simulink model "compare_filters"  (R2025a)
settings: Solver=VariableStepAuto  StartTime=0.0  StopTime=1.5  RelTol=1e-3
values from neighbouring files (symbols this model uses):
  phi_corr_LUT_param = Simulink.Parameter(phi_corr_LUT)    [lut_script.m]
undefined symbols (not defined in the file or in its folder): closed_loop, D_duty_cycle, D_m, DiscIntNeverNeededParam, hall_errors, I_duty_cycle, J_t, L_ss, lambda_m, P, P_duty_cycle, r_s, R_vs, T_m, theta_v, use_LUT, V_bus
libraries: spsMosfetLib x18, spsSeriesRLCBranchLib x12, spsVoltageMeasurementLib x9, spsControlledCurrentSourceLib x9, slpidlib x6, eeGeneralControl x3, simulink x3, embmathops x3, spsControlledVoltageSourceLib x3, spsPWMGeneratorDCDCLib x3, spsDCVoltageSourceLib x3, sps_lib x3
(part 1 of 3)
settings Model: Creator=rnashota.stu  LastModifiedBy=rnashota.stu

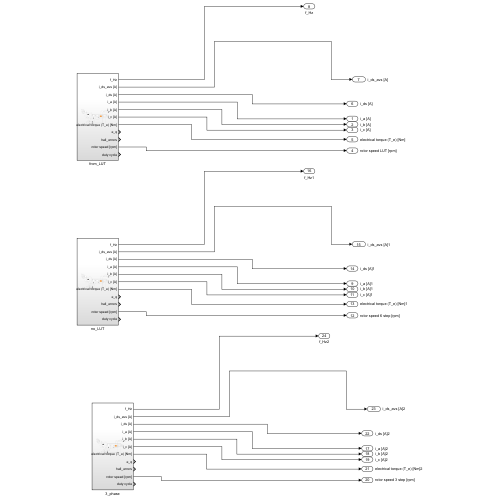
[thumbnail: Simulink's stored preview of the top-level diagram]
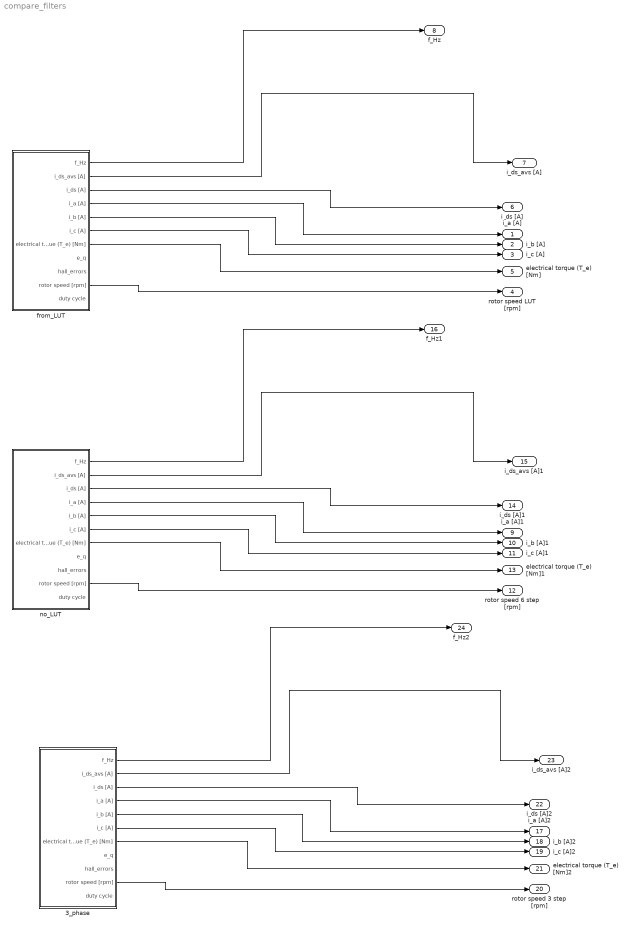
== system compare_filters ==
  3_phase : Subsystem
  from_LUT : Subsystem
  no_LUT : Subsystem
  i_a [A] : Outport
  i_b [A] : Outport  Port=2
  i_c [A] : Outport  Port=3
  rotor speed LUT [rpm] : Outport  Port=4
  electrical torque (T_e) [Nm] : Outport  Port=5
  i_ds [A] : Outport  Port=6
  i_ds_avs [A] : Outport  Port=7
  f_Hz : Outport  Port=8
  i_a [A]1 : Outport  Port=9
  i_b [A]1 : Outport  Port=10
  i_c [A]1 : Outport  Port=11
  rotor speed 6 step [rpm] : Outport  Port=12
  electrical torque (T_e) [Nm]1 : Outport  Port=13
  i_ds [A]1 : Outport  Port=14
  i_ds_avs [A]1 : Outport  Port=15
  f_Hz1 : Outport  Port=16
  i_a [A]2 : Outport  Port=17
  i_b [A]2 : Outport  Port=18
  i_c [A]2 : Outport  Port=19
  rotor speed 3 step [rpm] : Outport  Port=20
  electrical torque (T_e) [Nm]2 : Outport  Port=21
  i_ds [A]2 : Outport  Port=22
  i_ds_avs [A]2 : Outport  Port=23
  f_Hz2 : Outport  Port=24
  wires:
  from_LUT/1(f_Hz) -> f_Hz/1
  from_LUT/2(i_ds_avs [A]) -> i_ds_avs [A]/1
  from_LUT/3(i_ds [A]) -> i_ds [A]/1
  from_LUT/4(i_a [A]) -> i_a [A]/1
  from_LUT/5(i_b [A]) -> i_b [A]/1
  from_LUT/6(i_c [A]) -> i_c [A]/1
  from_LUT/7(electrical torque (T_e) [Nm]) -> electrical torque (T_e) [Nm]/1
  from_LUT/10(rotor speed [rpm]) -> rotor speed LUT [rpm]/1
  no_LUT/7(electrical torque (T_e) [Nm]) -> electrical torque (T_e) [Nm]1/1
  no_LUT/10(rotor speed [rpm]) -> rotor speed 6 step [rpm]/1
  no_LUT/2(i_ds_avs [A]) -> i_ds_avs [A]1/1
  no_LUT/3(i_ds [A]) -> i_ds [A]1/1
  no_LUT/6(i_c [A]) -> i_c [A]1/1
  no_LUT/1(f_Hz) -> f_Hz1/1
  no_LUT/4(i_a [A]) -> i_a [A]1/1
  no_LUT/5(i_b [A]) -> i_b [A]1/1
  3_phase/3(i_ds [A]) -> i_ds [A]2/1
  3_phase/5(i_b [A]) -> i_b [A]2/1
  3_phase/2(i_ds_avs [A]) -> i_ds_avs [A]2/1
  3_phase/6(i_c [A]) -> i_c [A]2/1
  3_phase/10(rotor speed [rpm]) -> rotor speed 3 step [rpm]/1
  3_phase/4(i_a [A]) -> i_a [A]2/1
  3_phase/1(f_Hz) -> f_Hz2/1
  3_phase/7(electrical torque (T_e) [Nm]) -> electrical torque (T_e) [Nm]2/1

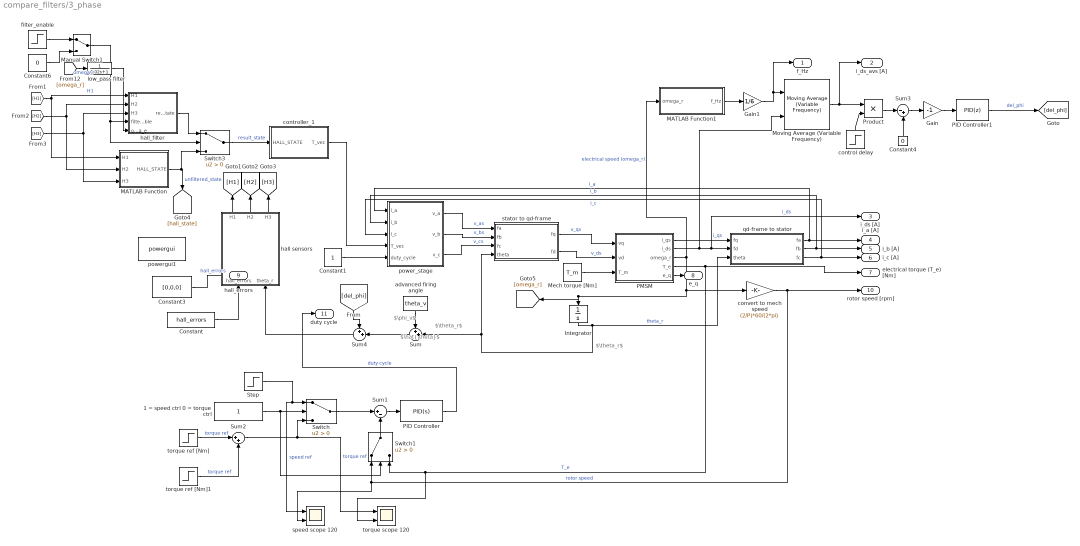
== system compare_filters/3_phase ==
  note: $\theta_r$
  note: $\hat{\theta}$
  note: $\phi_v$
  note: $\theta_r$
  1 = speed ctrl 0 = torque ctrl : Constant
  Constant : Constant  Value=hall_errors
  Constant1 : Constant
  Constant3 : Constant  Value=[0,0,0]
  Constant4 : Constant  Value=0
  Constant6 : Constant  Value=0
  Gain : Gain  Gain=-1
  Gain1 : Gain  Gain=1/6
  Integrator : Integrator
  MATLAB Function : MATLAB Function  TreatAsAtomicUnit=on
  MATLAB Function1 : MATLAB Function  TreatAsAtomicUnit=on
  Manual Switch1 : ManualSwitch
  Mech torque [Nm] : Constant  Value=T_m
  Moving Average (Variable Frequency) : eeGeneralControl/Moving Average (Variable Frequency)  VariantControl=Variant1  LabelModeActiveChoice=Continuous  f0=60  fmin=1  x0=0  BufferSize=32768  Ts=0
      settings: LibrarySourceBlock=|
      | ee_sl_lib/General Control/Moving Average
      | (Variable Frequency)
  PID Controller : slpidlib/PID Controller  Controller=PID  Form=Parallel  TimeDomain=Continuous-time  UseExternalTs=off  SampleTime=-1  IntegratorMethod=Forward Euler  FilterMethod=Forward Euler  ControllerParametersSource=internal  P=P_duty_cycle  I=I_duty_cycle  UseKiTs=off  D=D_duty_cycle  UseExternalDerivativeSource=off  N=100  UseFilter=on  TunerSelectOption=Transfer Function Based (PID Tuner App)  InitialConditionSource=internal  InitialConditionForIntegrator=0  InitialConditionForFilter=0  DifferentiatorICPrevScaledInput=0  ExternalReset=none  TrackingMode=off  Kt=1  LimitOutput=on  SatLimitsSource=internal  UpperSaturationLimit=1  LowerSaturationLimit=0  LinearizeAsGain=on  AntiWindupMode=none  Kb=1  LimitIntegrator=off  UpperIntegratorSaturationLimit=inf  LowerIntegratorSaturationLimit=-inf  POutMin=[]  POutMax=[]  IOutMin=[]  IOutMax=[]  DOutMin=[]  DOutMax=[]  NOutMin=[]  NOutMax=[]  SumOutMin=[]  SumOutMax=[]  SaturationOutMin=[]  SaturationOutMax=[]  PParamMin=[]  PParamMax=[]  IParamMin=[]  IParamMax=[]  DParamMin=[]  DParamMax=[]  NParamMin=[]  NParamMax=[]  KbParamMin=[]  KbParamMax=[]  KtParamMin=[]  KtParamMax=[]  KbOutMin=[]  KbOutMax=[]  KtOutMin=[]  KtOutMax=[]  IntegratorOutMin=[]  IntegratorOutMax=[]  FilterOutMin=[]  FilterOutMax=[]  SumI1OutMin=[]  SumI1OutMax=[]  SumI2OutMin=[]  SumI2OutMax=[]  SumI3OutMin=[]  SumI3OutMax=[]  SumI4OutMin=[]  SumI4OutMax=[]  SumDOutMin=[]  SumDOutMax=[]  DifferentiatorOutMin=[]  DifferentiatorOutMax=[]  FilterDiffOutCoefMin=[]  FilterDiffOutCoefMax=[]  ReciprocalOutMin=[]  ReciprocalOutMax=[]  SumDenOutMin=[]  SumDenOutMax=[]  SumNumOutMin=[]  SumNumOutMax=[]  DivideOutMin=[]  DivideOutMax=[]  UdiffTsProdOutMin=[]  UdiffTsProdOutMax=[]  NTsProdOutMin=[]  NTsProdOutMax=[]  UintegralTsProdOutMin=[]  UintegralTsProdOutMax=[]  UngainTsProdOutMin=[]  UngainTsProdOutMax=[]  ClampingZeroOutDataTypeStr=Inherit: Inherit via back propagation  ClampingZeroOutMin=[]  ClampingZeroOutMax=[]  FilterDenConstantOutDataTypeStr=Inherit: Inherit via back propagation  FilterDenConstantOutMin=[]  FilterDenConstantOutMax=[]  PCopyOutDataTypeStr=Inherit: Inherit via back propagation  PCopyOutMin=[]  PCopyOutMax=[]  NCopyOutDataTypeStr=Inherit: Inherit via back propagation  NCopyOutMin=[]  NCopyOutMax=[]  IntegratorContinuousStateAttributes=''  IntegratorStateMustResolveToSignalObject=off  IntegratorRTWStateStorageClass=Auto  FilterContinuousStateAttributes=''  FilterStateMustResolveToSignalObject=off  FilterRTWStateStorageClass=Auto  ParallelPVariant=InternalParameters  IdealPVariant=Disabled  IVariant=InternalParameters  DVariant=InternalParameters  IntegratorVariant=Continuous  SatVariant=Enabled  AWVariant=Passthrough  PCopyVariant=Disabled  TRVariant=Disabled  FdbkBlocksVariant=Forward  IdealPFdbkVariant=Disabled  SatFdbkVariant=Disabled  DerivativeFilterVariant=ContFilter  NVariant=InternalParameters  NCopyVariant=Disabled  FilterICVariant=InternalICsFilter  IntegratorICVariant=InternalICs  ExternalResetVariant=Disabled  TRSumVariant=Passthrough  SumFdbkVariant=Disabled  SumVariant=Sum_PID  TsampFilterVariant=InternalTs  TsampNgainVariant=Passthrough  TsampIntegralVariant=Disabled_SignalSpec  ExternalSaturationOutDataTypeStr=Inherit: Same as second input  DerivativeSourceVariant=ErrorSignal  PreIntVariant=InternalPreInt
  PID Controller1 : slpidlib/PID Controller  Controller=PID  Form=Parallel  TimeDomain=Discrete-time  UseExternalTs=off  SampleTime=-1  IntegratorMethod=Forward Euler  FilterMethod=Forward Euler  ControllerParametersSource=internal  P=0.0068  I=0.744  UseKiTs=off  D=0  UseExternalDerivativeSource=off  N=100  UseFilter=on  TunerSelectOption=Transfer Function Based (PID Tuner App)  InitialConditionSource=internal  InitialConditionForIntegrator=0  InitialConditionForFilter=0  DifferentiatorICPrevScaledInput=0  ExternalReset=none  TrackingMode=off  Kt=1  LimitOutput=on  SatLimitsSource=internal  UpperSaturationLimit=pi/3  LowerSaturationLimit=-pi/3  LinearizeAsGain=on  AntiWindupMode=none  Kb=1  LimitIntegrator=off  UpperIntegratorSaturationLimit=inf  LowerIntegratorSaturationLimit=-inf  POutMin=[]  POutMax=[]  IOutMin=[]  IOutMax=[]  DOutMin=[]  DOutMax=[]  NOutMin=[]  NOutMax=[]  SumOutMin=[]  SumOutMax=[]  SaturationOutMin=[]  SaturationOutMax=[]  PParamMin=[]  PParamMax=[]  IParamMin=[]  IParamMax=[]  DParamMin=[]  DParamMax=[]  NParamMin=[]  NParamMax=[]  KbParamMin=[]  KbParamMax=[]  KtParamMin=[]  KtParamMax=[]  KbOutMin=[]  KbOutMax=[]  KtOutMin=[]  KtOutMax=[]  IntegratorOutMin=[]  IntegratorOutMax=[]  FilterOutMin=[]  FilterOutMax=[]  SumI1OutMin=[]  SumI1OutMax=[]  SumI2OutMin=[]  SumI2OutMax=[]  SumI3OutMin=[]  SumI3OutMax=[]  SumI4OutMin=[]  SumI4OutMax=[]  SumDOutMin=[]  SumDOutMax=[]  DifferentiatorOutMin=[]  DifferentiatorOutMax=[]  FilterDiffOutCoefMin=[]  FilterDiffOutCoefMax=[]  ReciprocalOutMin=[]  ReciprocalOutMax=[]  SumDenOutMin=[]  SumDenOutMax=[]  SumNumOutMin=[]  SumNumOutMax=[]  DivideOutMin=[]  DivideOutMax=[]  UdiffTsProdOutMin=[]  UdiffTsProdOutMax=[]  NTsProdOutMin=[]  NTsProdOutMax=[]  UintegralTsProdOutMin=[]  UintegralTsProdOutMax=[]  UngainTsProdOutMin=[]  UngainTsProdOutMax=[]  ClampingZeroOutDataTypeStr=Inherit: Inherit via back propagation  ClampingZeroOutMin=[]  ClampingZeroOutMax=[]  FilterDenConstantOutDataTypeStr=Inherit: Inherit via back propagation  FilterDenConstantOutMin=[]  FilterDenConstantOutMax=[]  PCopyOutDataTypeStr=Inherit: Inherit via back propagation  PCopyOutMin=[]  PCopyOutMax=[]  NCopyOutDataTypeStr=Inherit: Inherit via back propagation  NCopyOutMin=[]  NCopyOutMax=[]  IntegratorContinuousStateAttributes=''  IntegratorStateMustResolveToSignalObject=off  IntegratorRTWStateStorageClass=Auto  FilterContinuousStateAttributes=''  FilterStateMustResolveToSignalObject=off  FilterRTWStateStorageClass=Auto  ParallelPVariant=InternalParameters  IdealPVariant=Disabled  IVariant=InternalParameters  DVariant=InternalParameters  IntegratorVariant=Discrete  SatVariant=Enabled  AWVariant=Passthrough  PCopyVariant=Disabled  TRVariant=Disabled  FdbkBlocksVariant=Forward  IdealPFdbkVariant=Disabled  SatFdbkVariant=Disabled  DerivativeFilterVariant=ForwardEulerFilter  NVariant=InternalParameters  NCopyVariant=Disabled  FilterICVariant=InternalICsFilter  IntegratorICVariant=InternalICs  ExternalResetVariant=Disabled  TRSumVariant=Passthrough  SumFdbkVariant=Disabled  SumVariant=Sum_PID  TsampFilterVariant=InternalTs  TsampNgainVariant=Passthrough  TsampIntegralVariant=Disabled_SignalSpec  ExternalSaturationOutDataTypeStr=Inherit: Same as second input  DerivativeSourceVariant=ErrorSignal  PreIntVariant=InternalPreInt
  PMSM : Subsystem
  Product : Product
  Step : Step  Time=0.1  After=1000  SampleTime=0
  Sum : Sum  Inputs=++|
  Sum1 : Sum  Inputs=|+-
  Sum2 : Sum  Inputs=|++
  Sum3 : Sum  Inputs=|-+
  Sum4 : Sum  Inputs=++|
  Switch : Switch  Criteria=u2 > Threshold  SaturateOnIntegerOverflow=off  InputSameDT=off
  Switch1 : Switch  Criteria=u2 > Threshold  SaturateOnIntegerOverflow=off  InputSameDT=off
  Switch3 : Switch  Criteria=u2 > Threshold  SaturateOnIntegerOverflow=off  InputSameDT=off
  advanced firing angle : Constant  Value=theta_v
  control delay : Step  Time=2  SampleTime=0
  controller_1 : MATLAB Function  TreatAsAtomicUnit=on
  convert to mech speed : Gain  Gain=(2/P)*60/(2*pi)
  filter_enable : Step  Time=0.5  SampleTime=0
  hall sensors : MATLAB Function  TreatAsAtomicUnit=on
  hall_filter : Subsystem
  low_pass filter : TransferFcn  Denominator=[0.02 1]
  power_stage : Subsystem
  powergui1 : sps_lib/powergui  Priority=1  SimulationMode=Discrete  SampleTime=1e-6  frequency=60  Iterations=50  frequencyindice=0  Pbase=100e6  ErrMax=1e-4  UnitsV=kV  UnitsW=MW  buscounter=0  FunctionMessages=off  echomessages=off  EnableUseOfTLC=off  CurrentSourceSwitches=off  DisableSnubberDevices=off  DisableRonSwitches=off  DisableVfSwitches=off  DisplayEquations=off  AutomaticDiscreteSolvers=off  SolverType=Tustin/Backward Euler (TBE)  Interpol=off  ExternalGateDelay=off  methode=off  Ts=100  x0status=blocks  SPID=on  SwTol=0  HookPort=off  NonlinearTolerance=1e-4  nMaxIteration=100  ContinueOnMaxIteration=off  RestoreLinks=warning  ResistiveCurrentMeasurement=off  Frange=[0:2:500]  Ylog=off  Xlog=on  ShowGrid=off  save=off  variable=ZData  structure=0  ZoomFFT=off  StartTime=0.0  cycles=1  DisplayStyle=1  fundamental=60  FreqAxis=off  MaxFrequency=1000  frequencyindicesteady=1  RmsSteady=1  display=off
  qd-frame to stator : MATLAB Function  TreatAsAtomicUnit=on
  speed scope 120 : Scope  NumInputPorts=2
      settings: ActiveDisplayYMinimum=-1.1385486491945782E+15  ActiveDisplayYMaximum=1.0246937842751196E+16  DataLoggingVariableName=ScopeData5
  stator to qd-frame : MATLAB Function  TreatAsAtomicUnit=on
  torque ref [Nm] : Step  Time=0.1  After=1e-1  SampleTime=0  ZeroCross=off
  torque ref [Nm]1 : Step  After=-0.5e-1  SampleTime=0
  torque scope 120 : Scope  NumInputPorts=2
      settings: ActiveDisplayYMinimum=-0.89883  ActiveDisplayYMaximum=8.08945  DataLoggingVariableName=ScopeData6
  f_Hz : Outport
  i_ds_avs [A] : Outport  Port=2
  i_ds [A] : Outport  Port=3
  i_a [A] : Outport  Port=4
  i_b [A] : Outport  Port=5
  i_c [A] : Outport  Port=6
  electrical torque (T_e) [Nm] : Outport  Port=7
  e_q : Outport  Port=8
  hall_errors : Outport  Port=9
  rotor speed [rpm] : Outport  Port=10
  duty cycle : Outport  Port=11
  wires:
  Sum1/1 -> PID Controller/1
  Sum3/1 -> Gain/1
  power_stage/1(v_a) -> stator to qd-frame/1(fa)  "v_as"
  hall sensors/3(H3) -> [H3]
  qd-frame to stator/1(fa) -> i_a [A]/1, power_stage/1(i_a)  "i_a"
  convert to mech speed/1 -> rotor speed [rpm]/1, Switch1/1, speed scope 120/2  "rotor speed"
  qd-frame to stator/2(fb) -> i_b [A]/1, power_stage/2(i_b)  "i_b"
  hall_filter/1(result_state) -> Switch3/1
  PMSM/3(omega_r) -> MATLAB Function1/1(omega_r), convert to mech speed/1, [omega_r], Integrator/1  "electrical speed (omega_r)"
  MATLAB Function/1(HALL_STATE) -> [hall_state], Switch3/3  "unfiltered_state"
  Constant6/1 -> Manual Switch1/2
  Sum2/1 -> torque scope 120/1, Switch/3  "torque ref"
  control delay/1 -> Product/2
  [H1] -> hall_filter/1(H1), MATLAB Function/1(H1)  "H1"
  Mech torque [Nm]/1 -> PMSM/3(T_m)
  Step/1 -> speed scope 120/1, Switch/1  "speed ref"
  Switch3/1 -> controller_1/1(HALL_STATE)  "result_state"
  PMSM/2(i_ds) -> i_ds [A]/1, qd-frame to stator/2(fd), Moving Average (Variable Frequency)/2  "i_ds"
  Constant/1 -> hall sensors/1(hall_errors)
  PMSM/1(i_qs) -> qd-frame to stator/1(fq)  "i_qs"
  [omega_r] -> low_pass filter/1  "omega_r"
  power_stage/2(v_b) -> stator to qd-frame/2(fb)  "v_bs"
  Constant1/1 -> power_stage/5(duty_cycle)
  Manual Switch1/1 -> Switch3/2, hall_filter/4(filter_enable)
  PID Controller1/1 -> [del_phi]  "del_phi"
  hall sensors/1(H1) -> [H1]
  1 = speed ctrl 0 = torque ctrl/1 -> Switch/2, Switch1/2
  PMSM/4(T_e) -> electrical torque (T_e) [Nm]/1, torque scope 120/2, Switch1/3  "T_e"
  Moving Average (Variable Frequency)/1 -> i_ds_avs [A]/1, Product/1
  [H2] -> hall_filter/2(H2), MATLAB Function/2(H2)
  PMSM/5(e_q) -> e_q/1
  MATLAB Function1/1(f_Hz) -> Gain1/1
  torque ref [Nm]/1 -> Sum2/1  "torque ref"
  hall sensors/2(H2) -> [H2]
  Sum4/1 -> hall sensors/2(theta_r)
  Gain/1 -> PID Controller1/1
  filter_enable/1 -> Manual Switch1/1
  low_pass filter/1 -> hall_filter/5(omega_e)
  Constant3/1 -> hall_errors/1  "hall_errors"
  power_stage/3(v_c) -> stator to qd-frame/3(fc)  "v_cs"
  [del_phi] -> Sum4/1
  qd-frame to stator/3(fc) -> i_c [A]/1, power_stage/3(i_c)  "i_c"
  torque ref [Nm]1/1 -> Sum2/2  "torque ref"
  Switch1/1 -> Sum1/2
  Product/1 -> Sum3/1
  Integrator/1 -> stator to qd-frame/4(theta), Sum/2, qd-frame to stator/3(theta)  "theta_r"
  PID Controller/1 -> duty cycle/1  "duty cycle"
  Constant4/1 -> Sum3/2
  Gain1/1 -> f_Hz/1, Moving Average (Variable Frequency)/1
  stator to qd-frame/1(fq) -> PMSM/1(vq)  "v_qs"
  Sum/1 -> Sum4/2
  Switch/1 -> Sum1/1
  [H3] -> hall_filter/3(H3), MATLAB Function/3(H3)
  advanced firing angle/1 -> Sum/1
  stator to qd-frame/2(fd) -> PMSM/2(vd)  "v_ds"
  controller_1/1(T_vec) -> power_stage/4(T_vec)

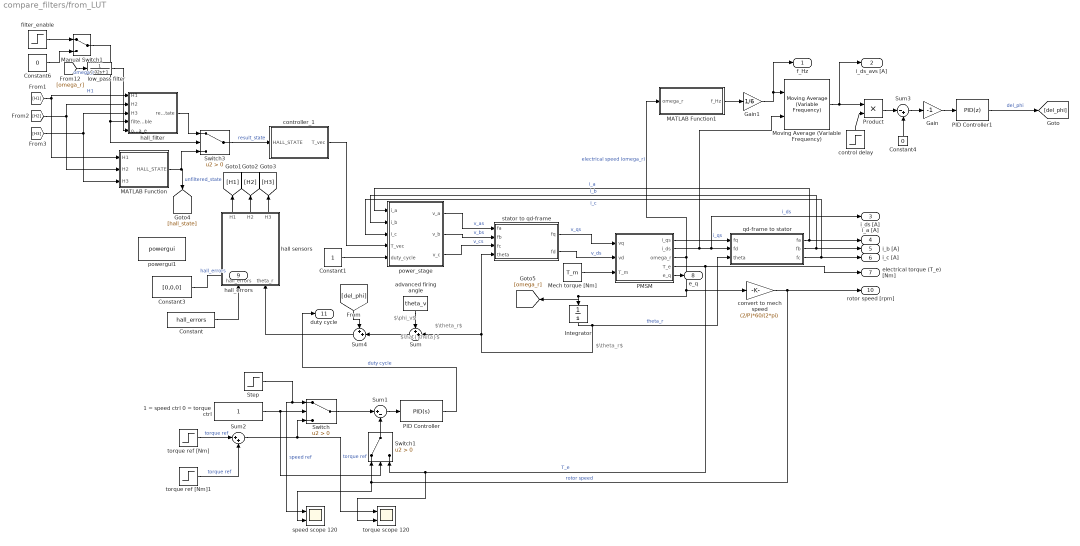
== system compare_filters/from_LUT ==
  note: $\theta_r$
  note: $\hat{\theta}$
  note: $\phi_v$
  note: $\theta_r$
  1 = speed ctrl 0 = torque ctrl : Constant
  Constant : Constant  Value=hall_errors
  Constant1 : Constant
  Constant3 : Constant  Value=[0,0,0]
  Constant4 : Constant  Value=0
  Constant6 : Constant  Value=0
  Gain : Gain  Gain=-1
  Gain1 : Gain  Gain=1/6
  Integrator : Integrator
  MATLAB Function : MATLAB Function  TreatAsAtomicUnit=on
  MATLAB Function1 : MATLAB Function  TreatAsAtomicUnit=on
  Manual Switch1 : ManualSwitch
  Mech torque [Nm] : Constant  Value=T_m
  Moving Average (Variable Frequency) : eeGeneralControl/Moving Average (Variable Frequency)  VariantControl=Variant1  LabelModeActiveChoice=Continuous  f0=60  fmin=1  x0=0  BufferSize=32768  Ts=0
      settings: LibrarySourceBlock=|
      | ee_sl_lib/General Control/Moving Average
      | (Variable Frequency)
  PID Controller : slpidlib/PID Controller  Controller=PID  Form=Parallel  TimeDomain=Continuous-time  UseExternalTs=off  SampleTime=-1  IntegratorMethod=Forward Euler  FilterMethod=Forward Euler  ControllerParametersSource=internal  P=P_duty_cycle  I=I_duty_cycle  UseKiTs=off  D=D_duty_cycle  UseExternalDerivativeSource=off  N=100  UseFilter=on  TunerSelectOption=Transfer Function Based (PID Tuner App)  InitialConditionSource=internal  InitialConditionForIntegrator=0  InitialConditionForFilter=0  DifferentiatorICPrevScaledInput=0  ExternalReset=none  TrackingMode=off  Kt=1  LimitOutput=on  SatLimitsSource=internal  UpperSaturationLimit=1  LowerSaturationLimit=0  LinearizeAsGain=on  AntiWindupMode=none  Kb=1  LimitIntegrator=off  UpperIntegratorSaturationLimit=inf  LowerIntegratorSaturationLimit=-inf  POutMin=[]  POutMax=[]  IOutMin=[]  IOutMax=[]  DOutMin=[]  DOutMax=[]  NOutMin=[]  NOutMax=[]  SumOutMin=[]  SumOutMax=[]  SaturationOutMin=[]  SaturationOutMax=[]  PParamMin=[]  PParamMax=[]  IParamMin=[]  IParamMax=[]  DParamMin=[]  DParamMax=[]  NParamMin=[]  NParamMax=[]  KbParamMin=[]  KbParamMax=[]  KtParamMin=[]  KtParamMax=[]  KbOutMin=[]  KbOutMax=[]  KtOutMin=[]  KtOutMax=[]  IntegratorOutMin=[]  IntegratorOutMax=[]  FilterOutMin=[]  FilterOutMax=[]  SumI1OutMin=[]  SumI1OutMax=[]  SumI2OutMin=[]  SumI2OutMax=[]  SumI3OutMin=[]  SumI3OutMax=[]  SumI4OutMin=[]  SumI4OutMax=[]  SumDOutMin=[]  SumDOutMax=[]  DifferentiatorOutMin=[]  DifferentiatorOutMax=[]  FilterDiffOutCoefMin=[]  FilterDiffOutCoefMax=[]  ReciprocalOutMin=[]  ReciprocalOutMax=[]  SumDenOutMin=[]  SumDenOutMax=[]  SumNumOutMin=[]  SumNumOutMax=[]  DivideOutMin=[]  DivideOutMax=[]  UdiffTsProdOutMin=[]  UdiffTsProdOutMax=[]  NTsProdOutMin=[]  NTsProdOutMax=[]  UintegralTsProdOutMin=[]  UintegralTsProdOutMax=[]  UngainTsProdOutMin=[]  UngainTsProdOutMax=[]  ClampingZeroOutDataTypeStr=Inherit: Inherit via back propagation  ClampingZeroOutMin=[]  ClampingZeroOutMax=[]  FilterDenConstantOutDataTypeStr=Inherit: Inherit via back propagation  FilterDenConstantOutMin=[]  FilterDenConstantOutMax=[]  PCopyOutDataTypeStr=Inherit: Inherit via back propagation  PCopyOutMin=[]  PCopyOutMax=[]  NCopyOutDataTypeStr=Inherit: Inherit via back propagation  NCopyOutMin=[]  NCopyOutMax=[]  IntegratorContinuousStateAttributes=''  IntegratorStateMustResolveToSignalObject=off  IntegratorRTWStateStorageClass=Auto  FilterContinuousStateAttributes=''  FilterStateMustResolveToSignalObject=off  FilterRTWStateStorageClass=Auto  ParallelPVariant=InternalParameters  IdealPVariant=Disabled  IVariant=InternalParameters  DVariant=InternalParameters  IntegratorVariant=Continuous  SatVariant=Enabled  AWVariant=Passthrough  PCopyVariant=Disabled  TRVariant=Disabled  FdbkBlocksVariant=Forward  IdealPFdbkVariant=Disabled  SatFdbkVariant=Disabled  DerivativeFilterVariant=ContFilter  NVariant=InternalParameters  NCopyVariant=Disabled  FilterICVariant=InternalICsFilter  IntegratorICVariant=InternalICs  ExternalResetVariant=Disabled  TRSumVariant=Passthrough  SumFdbkVariant=Disabled  SumVariant=Sum_PID  TsampFilterVariant=InternalTs  TsampNgainVariant=Passthrough  TsampIntegralVariant=Disabled_SignalSpec  ExternalSaturationOutDataTypeStr=Inherit: Same as second input  DerivativeSourceVariant=ErrorSignal  PreIntVariant=InternalPreInt
  PID Controller1 : slpidlib/PID Controller  Controller=PID  Form=Parallel  TimeDomain=Discrete-time  UseExternalTs=off  SampleTime=-1  IntegratorMethod=Forward Euler  FilterMethod=Forward Euler  ControllerParametersSource=internal  P=0.0068  I=0.744  UseKiTs=off  D=0  UseExternalDerivativeSource=off  N=100  UseFilter=on  TunerSelectOption=Transfer Function Based (PID Tuner App)  InitialConditionSource=internal  InitialConditionForIntegrator=0  InitialConditionForFilter=0  DifferentiatorICPrevScaledInput=0  ExternalReset=none  TrackingMode=off  Kt=1  LimitOutput=on  SatLimitsSource=internal  UpperSaturationLimit=pi/3  LowerSaturationLimit=-pi/3  LinearizeAsGain=on  AntiWindupMode=none  Kb=1  LimitIntegrator=off  UpperIntegratorSaturationLimit=inf  LowerIntegratorSaturationLimit=-inf  POutMin=[]  POutMax=[]  IOutMin=[]  IOutMax=[]  DOutMin=[]  DOutMax=[]  NOutMin=[]  NOutMax=[]  SumOutMin=[]  SumOutMax=[]  SaturationOutMin=[]  SaturationOutMax=[]  PParamMin=[]  PParamMax=[]  IParamMin=[]  IParamMax=[]  DParamMin=[]  DParamMax=[]  NParamMin=[]  NParamMax=[]  KbParamMin=[]  KbParamMax=[]  KtParamMin=[]  KtParamMax=[]  KbOutMin=[]  KbOutMax=[]  KtOutMin=[]  KtOutMax=[]  IntegratorOutMin=[]  IntegratorOutMax=[]  FilterOutMin=[]  FilterOutMax=[]  SumI1OutMin=[]  SumI1OutMax=[]  SumI2OutMin=[]  SumI2OutMax=[]  SumI3OutMin=[]  SumI3OutMax=[]  SumI4OutMin=[]  SumI4OutMax=[]  SumDOutMin=[]  SumDOutMax=[]  DifferentiatorOutMin=[]  DifferentiatorOutMax=[]  FilterDiffOutCoefMin=[]  FilterDiffOutCoefMax=[]  ReciprocalOutMin=[]  ReciprocalOutMax=[]  SumDenOutMin=[]  SumDenOutMax=[]  SumNumOutMin=[]  SumNumOutMax=[]  DivideOutMin=[]  DivideOutMax=[]  UdiffTsProdOutMin=[]  UdiffTsProdOutMax=[]  NTsProdOutMin=[]  NTsProdOutMax=[]  UintegralTsProdOutMin=[]  UintegralTsProdOutMax=[]  UngainTsProdOutMin=[]  UngainTsProdOutMax=[]  ClampingZeroOutDataTypeStr=Inherit: Inherit via back propagation  ClampingZeroOutMin=[]  ClampingZeroOutMax=[]  FilterDenConstantOutDataTypeStr=Inherit: Inherit via back propagation  FilterDenConstantOutMin=[]  FilterDenConstantOutMax=[]  PCopyOutDataTypeStr=Inherit: Inherit via back propagation  PCopyOutMin=[]  PCopyOutMax=[]  NCopyOutDataTypeStr=Inherit: Inherit via back propagation  NCopyOutMin=[]  NCopyOutMax=[]  IntegratorContinuousStateAttributes=''  IntegratorStateMustResolveToSignalObject=off  IntegratorRTWStateStorageClass=Auto  FilterContinuousStateAttributes=''  FilterStateMustResolveToSignalObject=off  FilterRTWStateStorageClass=Auto  ParallelPVariant=InternalParameters  IdealPVariant=Disabled  IVariant=InternalParameters  DVariant=InternalParameters  IntegratorVariant=Discrete  SatVariant=Enabled  AWVariant=Passthrough  PCopyVariant=Disabled  TRVariant=Disabled  FdbkBlocksVariant=Forward  IdealPFdbkVariant=Disabled  SatFdbkVariant=Disabled  DerivativeFilterVariant=ForwardEulerFilter  NVariant=InternalParameters  NCopyVariant=Disabled  FilterICVariant=InternalICsFilter  IntegratorICVariant=InternalICs  ExternalResetVariant=Disabled  TRSumVariant=Passthrough  SumFdbkVariant=Disabled  SumVariant=Sum_PID  TsampFilterVariant=InternalTs  TsampNgainVariant=Passthrough  TsampIntegralVariant=Disabled_SignalSpec  ExternalSaturationOutDataTypeStr=Inherit: Same as second input  DerivativeSourceVariant=ErrorSignal  PreIntVariant=InternalPreInt
  PMSM : Subsystem
  Product : Product
  Step : Step  Time=0.1  After=1000  SampleTime=0
  Sum : Sum  Inputs=++|
  Sum1 : Sum  Inputs=|+-
  Sum2 : Sum  Inputs=|++
  Sum3 : Sum  Inputs=|-+
  Sum4 : Sum  Inputs=++|
  Switch : Switch  Criteria=u2 > Threshold  SaturateOnIntegerOverflow=off  InputSameDT=off
  Switch1 : Switch  Criteria=u2 > Threshold  SaturateOnIntegerOverflow=off  InputSameDT=off
  Switch3 : Switch  Criteria=u2 > Threshold  SaturateOnIntegerOverflow=off  InputSameDT=off
  advanced firing angle : Constant  Value=theta_v
  control delay : Step  Time=2  SampleTime=0
  controller_1 : MATLAB Function  TreatAsAtomicUnit=on
  convert to mech speed : Gain  Gain=(2/P)*60/(2*pi)
  filter_enable : Step  Time=0.5  SampleTime=0
  hall sensors : MATLAB Function  TreatAsAtomicUnit=on
  hall_filter : Subsystem
  low_pass filter : TransferFcn  Denominator=[0.02 1]
  power_stage : Subsystem
  powergui1 : sps_lib/powergui  Priority=1  SimulationMode=Discrete  SampleTime=1e-6  frequency=60  Iterations=50  frequencyindice=0  Pbase=100e6  ErrMax=1e-4  UnitsV=kV  UnitsW=MW  buscounter=0  FunctionMessages=off  echomessages=off  EnableUseOfTLC=off  CurrentSourceSwitches=off  DisableSnubberDevices=off  DisableRonSwitches=off  DisableVfSwitches=off  DisplayEquations=off  AutomaticDiscreteSolvers=off  SolverType=Tustin/Backward Euler (TBE)  Interpol=off  ExternalGateDelay=off  methode=off  Ts=100  x0status=blocks  SPID=on  SwTol=0  HookPort=off  NonlinearTolerance=1e-4  nMaxIteration=100  ContinueOnMaxIteration=off  RestoreLinks=warning  ResistiveCurrentMeasurement=off  Frange=[0:2:500]  Ylog=off  Xlog=on  ShowGrid=off  save=off  variable=ZData  structure=0  ZoomFFT=off  StartTime=0.0  cycles=1  DisplayStyle=1  fundamental=60  FreqAxis=off  MaxFrequency=1000  frequencyindicesteady=1  RmsSteady=1  display=off
  qd-frame to stator : MATLAB Function  TreatAsAtomicUnit=on
  speed scope 120 : Scope  NumInputPorts=2
      settings: ActiveDisplayYMinimum=-1.1385486491945782E+15  ActiveDisplayYMaximum=1.0246937842751196E+16  DataLoggingVariableName=ScopeData5
  stator to qd-frame : MATLAB Function  TreatAsAtomicUnit=on
  torque ref [Nm] : Step  Time=0.1  After=1e-1  SampleTime=0  ZeroCross=off
  torque ref [Nm]1 : Step  After=-0.5e-1  SampleTime=0
  torque scope 120 : Scope  NumInputPorts=2
      settings: ActiveDisplayYMinimum=-0.89883  ActiveDisplayYMaximum=8.08945  DataLoggingVariableName=ScopeData6
  f_Hz : Outport
  i_ds_avs [A] : Outport  Port=2
  i_ds [A] : Outport  Port=3
  i_a [A] : Outport  Port=4
  i_b [A] : Outport  Port=5
  i_c [A] : Outport  Port=6
  electrical torque (T_e) [Nm] : Outport  Port=7
  e_q : Outport  Port=8
  hall_errors : Outport  Port=9
  rotor speed [rpm] : Outport  Port=10
  duty cycle : Outport  Port=11
  wires:
  Sum1/1 -> PID Controller/1
  Sum3/1 -> Gain/1
  power_stage/1(v_a) -> stator to qd-frame/1(fa)  "v_as"
  hall sensors/3(H3) -> [H3]
  qd-frame to stator/1(fa) -> i_a [A]/1, power_stage/1(i_a)  "i_a"
  convert to mech speed/1 -> rotor speed [rpm]/1, Switch1/1, speed scope 120/2  "rotor speed"
  qd-frame to stator/2(fb) -> i_b [A]/1, power_stage/2(i_b)  "i_b"
  hall_filter/1(result_state) -> Switch3/1
  PMSM/3(omega_r) -> MATLAB Function1/1(omega_r), convert to mech speed/1, [omega_r], Integrator/1  "electrical speed (omega_r)"
  MATLAB Function/1(HALL_STATE) -> [hall_state], Switch3/3  "unfiltered_state"
  Constant6/1 -> Manual Switch1/2
  Sum2/1 -> torque scope 120/1, Switch/3  "torque ref"
  control delay/1 -> Product/2
  [H1] -> hall_filter/1(H1), MATLAB Function/1(H1)  "H1"
  Mech torque [Nm]/1 -> PMSM/3(T_m)
  Step/1 -> speed scope 120/1, Switch/1  "speed ref"
  Switch3/1 -> controller_1/1(HALL_STATE)  "result_state"
  PMSM/2(i_ds) -> i_ds [A]/1, qd-frame to stator/2(fd), Moving Average (Variable Frequency)/2  "i_ds"
  Constant/1 -> hall sensors/1(hall_errors)
  PMSM/1(i_qs) -> qd-frame to stator/1(fq)  "i_qs"
  [omega_r] -> low_pass filter/1  "omega_r"
  power_stage/2(v_b) -> stator to qd-frame/2(fb)  "v_bs"
  Constant1/1 -> power_stage/5(duty_cycle)
  Manual Switch1/1 -> Switch3/2, hall_filter/4(filter_enable)
  PID Controller1/1 -> [del_phi]  "del_phi"
  hall sensors/1(H1) -> [H1]
  1 = speed ctrl 0 = torque ctrl/1 -> Switch/2, Switch1/2
  PMSM/4(T_e) -> electrical torque (T_e) [Nm]/1, torque scope 120/2, Switch1/3  "T_e"
  Moving Average (Variable Frequency)/1 -> i_ds_avs [A]/1, Product/1
  [H2] -> hall_filter/2(H2), MATLAB Function/2(H2)
  PMSM/5(e_q) -> e_q/1
  MATLAB Function1/1(f_Hz) -> Gain1/1
  torque ref [Nm]/1 -> Sum2/1  "torque ref"
  hall sensors/2(H2) -> [H2]
  Sum4/1 -> hall sensors/2(theta_r)
  Gain/1 -> PID Controller1/1
  filter_enable/1 -> Manual Switch1/1
  low_pass filter/1 -> hall_filter/5(omega_e)
  Constant3/1 -> hall_errors/1  "hall_errors"
  power_stage/3(v_c) -> stator to qd-frame/3(fc)  "v_cs"
  [del_phi] -> Sum4/1
  qd-frame to stator/3(fc) -> i_c [A]/1, power_stage/3(i_c)  "i_c"
  torque ref [Nm]1/1 -> Sum2/2  "torque ref"
  Switch1/1 -> Sum1/2
  Product/1 -> Sum3/1
  Integrator/1 -> stator to qd-frame/4(theta), Sum/2, qd-frame to stator/3(theta)  "theta_r"
  PID Controller/1 -> duty cycle/1  "duty cycle"
  Constant4/1 -> Sum3/2
  Gain1/1 -> f_Hz/1, Moving Average (Variable Frequency)/1
  stator to qd-frame/1(fq) -> PMSM/1(vq)  "v_qs"
  Sum/1 -> Sum4/2
  Switch/1 -> Sum1/1
  [H3] -> hall_filter/3(H3), MATLAB Function/3(H3)
  advanced firing angle/1 -> Sum/1
  stator to qd-frame/2(fd) -> PMSM/2(vd)  "v_ds"
  controller_1/1(T_vec) -> power_stage/4(T_vec)

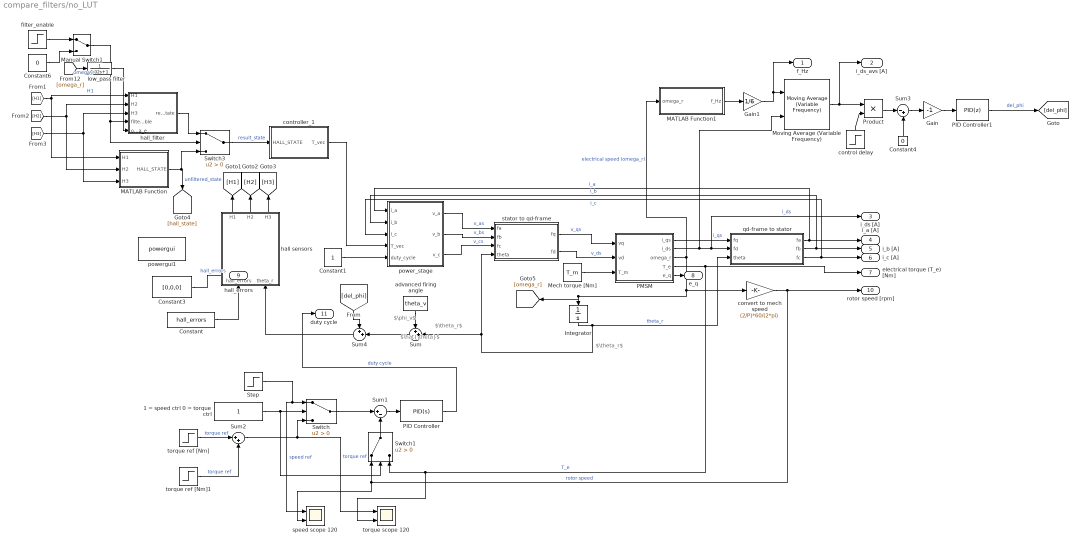
== system compare_filters/no_LUT ==
  note: $\theta_r$
  note: $\hat{\theta}$
  note: $\phi_v$
  note: $\theta_r$
  1 = speed ctrl 0 = torque ctrl : Constant
  Constant : Constant  Value=hall_errors
  Constant1 : Constant
  Constant3 : Constant  Value=[0,0,0]
  Constant4 : Constant  Value=0
  Constant6 : Constant  Value=0
  Gain : Gain  Gain=-1
  Gain1 : Gain  Gain=1/6
  Integrator : Integrator
  MATLAB Function : MATLAB Function  TreatAsAtomicUnit=on
  MATLAB Function1 : MATLAB Function  TreatAsAtomicUnit=on
  Manual Switch1 : ManualSwitch
  Mech torque [Nm] : Constant  Value=T_m
  Moving Average (Variable Frequency) : eeGeneralControl/Moving Average (Variable Frequency)  VariantControl=Variant1  LabelModeActiveChoice=Continuous  f0=60  fmin=1  x0=0  BufferSize=32768  Ts=0
      settings: LibrarySourceBlock=|
      | ee_sl_lib/General Control/Moving Average
      | (Variable Frequency)
  PID Controller : slpidlib/PID Controller  Controller=PID  Form=Parallel  TimeDomain=Continuous-time  UseExternalTs=off  SampleTime=-1  IntegratorMethod=Forward Euler  FilterMethod=Forward Euler  ControllerParametersSource=internal  P=P_duty_cycle  I=I_duty_cycle  UseKiTs=off  D=D_duty_cycle  UseExternalDerivativeSource=off  N=100  UseFilter=on  TunerSelectOption=Transfer Function Based (PID Tuner App)  InitialConditionSource=internal  InitialConditionForIntegrator=0  InitialConditionForFilter=0  DifferentiatorICPrevScaledInput=0  ExternalReset=none  TrackingMode=off  Kt=1  LimitOutput=on  SatLimitsSource=internal  UpperSaturationLimit=1  LowerSaturationLimit=0  LinearizeAsGain=on  AntiWindupMode=none  Kb=1  LimitIntegrator=off  UpperIntegratorSaturationLimit=inf  LowerIntegratorSaturationLimit=-inf  POutMin=[]  POutMax=[]  IOutMin=[]  IOutMax=[]  DOutMin=[]  DOutMax=[]  NOutMin=[]  NOutMax=[]  SumOutMin=[]  SumOutMax=[]  SaturationOutMin=[]  SaturationOutMax=[]  PParamMin=[]  PParamMax=[]  IParamMin=[]  IParamMax=[]  DParamMin=[]  DParamMax=[]  NParamMin=[]  NParamMax=[]  KbParamMin=[]  KbParamMax=[]  KtParamMin=[]  KtParamMax=[]  KbOutMin=[]  KbOutMax=[]  KtOutMin=[]  KtOutMax=[]  IntegratorOutMin=[]  IntegratorOutMax=[]  FilterOutMin=[]  FilterOutMax=[]  SumI1OutMin=[]  SumI1OutMax=[]  SumI2OutMin=[]  SumI2OutMax=[]  SumI3OutMin=[]  SumI3OutMax=[]  SumI4OutMin=[]  SumI4OutMax=[]  SumDOutMin=[]  SumDOutMax=[]  DifferentiatorOutMin=[]  DifferentiatorOutMax=[]  FilterDiffOutCoefMin=[]  FilterDiffOutCoefMax=[]  ReciprocalOutMin=[]  ReciprocalOutMax=[]  SumDenOutMin=[]  SumDenOutMax=[]  SumNumOutMin=[]  SumNumOutMax=[]  DivideOutMin=[]  DivideOutMax=[]  UdiffTsProdOutMin=[]  UdiffTsProdOutMax=[]  NTsProdOutMin=[]  NTsProdOutMax=[]  UintegralTsProdOutMin=[]  UintegralTsProdOutMax=[]  UngainTsProdOutMin=[]  UngainTsProdOutMax=[]  ClampingZeroOutDataTypeStr=Inherit: Inherit via back propagation  ClampingZeroOutMin=[]  ClampingZeroOutMax=[]  FilterDenConstantOutDataTypeStr=Inherit: Inherit via back propagation  FilterDenConstantOutMin=[]  FilterDenConstantOutMax=[]  PCopyOutDataTypeStr=Inherit: Inherit via back propagation  PCopyOutMin=[]  PCopyOutMax=[]  NCopyOutDataTypeStr=Inherit: Inherit via back propagation  NCopyOutMin=[]  NCopyOutMax=[]  IntegratorContinuousStateAttributes=''  IntegratorStateMustResolveToSignalObject=off  IntegratorRTWStateStorageClass=Auto  FilterContinuousStateAttributes=''  FilterStateMustResolveToSignalObject=off  FilterRTWStateStorageClass=Auto  ParallelPVariant=InternalParameters  IdealPVariant=Disabled  IVariant=InternalParameters  DVariant=InternalParameters  IntegratorVariant=Continuous  SatVariant=Enabled  AWVariant=Passthrough  PCopyVariant=Disabled  TRVariant=Disabled  FdbkBlocksVariant=Forward  IdealPFdbkVariant=Disabled  SatFdbkVariant=Disabled  DerivativeFilterVariant=ContFilter  NVariant=InternalParameters  NCopyVariant=Disabled  FilterICVariant=InternalICsFilter  IntegratorICVariant=InternalICs  ExternalResetVariant=Disabled  TRSumVariant=Passthrough  SumFdbkVariant=Disabled  SumVariant=Sum_PID  TsampFilterVariant=InternalTs  TsampNgainVariant=Passthrough  TsampIntegralVariant=Disabled_SignalSpec  ExternalSaturationOutDataTypeStr=Inherit: Same as second input  DerivativeSourceVariant=ErrorSignal  PreIntVariant=InternalPreInt
  PID Controller1 : slpidlib/PID Controller  Controller=PID  Form=Parallel  TimeDomain=Discrete-time  UseExternalTs=off  SampleTime=-1  IntegratorMethod=Forward Euler  FilterMethod=Forward Euler  ControllerParametersSource=internal  P=0.0068  I=0.744  UseKiTs=off  D=0  UseExternalDerivativeSource=off  N=100  UseFilter=on  TunerSelectOption=Transfer Function Based (PID Tuner App)  InitialConditionSource=internal  InitialConditionForIntegrator=0  InitialConditionForFilter=0  DifferentiatorICPrevScaledInput=0  ExternalReset=none  TrackingMode=off  Kt=1  LimitOutput=on  SatLimitsSource=internal  UpperSaturationLimit=pi/3  LowerSaturationLimit=-pi/3  LinearizeAsGain=on  AntiWindupMode=none  Kb=1  LimitIntegrator=off  UpperIntegratorSaturationLimit=inf  LowerIntegratorSaturationLimit=-inf  POutMin=[]  POutMax=[]  IOutMin=[]  IOutMax=[]  DOutMin=[]  DOutMax=[]  NOutMin=[]  NOutMax=[]  SumOutMin=[]  SumOutMax=[]  SaturationOutMin=[]  SaturationOutMax=[]  PParamMin=[]  PParamMax=[]  IParamMin=[]  IParamMax=[]  DParamMin=[]  DParamMax=[]  NParamMin=[]  NParamMax=[]  KbParamMin=[]  KbParamMax=[]  KtParamMin=[]  KtParamMax=[]  KbOutMin=[]  KbOutMax=[]  KtOutMin=[]  KtOutMax=[]  IntegratorOutMin=[]  IntegratorOutMax=[]  FilterOutMin=[]  FilterOutMax=[]  SumI1OutMin=[]  SumI1OutMax=[]  SumI2OutMin=[]  SumI2OutMax=[]  SumI3OutMin=[]  SumI3OutMax=[]  SumI4OutMin=[]  SumI4OutMax=[]  SumDOutMin=[]  SumDOutMax=[]  DifferentiatorOutMin=[]  DifferentiatorOutMax=[]  FilterDiffOutCoefMin=[]  FilterDiffOutCoefMax=[]  ReciprocalOutMin=[]  ReciprocalOutMax=[]  SumDenOutMin=[]  SumDenOutMax=[]  SumNumOutMin=[]  SumNumOutMax=[]  DivideOutMin=[]  DivideOutMax=[]  UdiffTsProdOutMin=[]  UdiffTsProdOutMax=[]  NTsProdOutMin=[]  NTsProdOutMax=[]  UintegralTsProdOutMin=[]  UintegralTsProdOutMax=[]  UngainTsProdOutMin=[]  UngainTsProdOutMax=[]  ClampingZeroOutDataTypeStr=Inherit: Inherit via back propagation  ClampingZeroOutMin=[]  ClampingZeroOutMax=[]  FilterDenConstantOutDataTypeStr=Inherit: Inherit via back propagation  FilterDenConstantOutMin=[]  FilterDenConstantOutMax=[]  PCopyOutDataTypeStr=Inherit: Inherit via back propagation  PCopyOutMin=[]  PCopyOutMax=[]  NCopyOutDataTypeStr=Inherit: Inherit via back propagation  NCopyOutMin=[]  NCopyOutMax=[]  IntegratorContinuousStateAttributes=''  IntegratorStateMustResolveToSignalObject=off  IntegratorRTWStateStorageClass=Auto  FilterContinuousStateAttributes=''  FilterStateMustResolveToSignalObject=off  FilterRTWStateStorageClass=Auto  ParallelPVariant=InternalParameters  IdealPVariant=Disabled  IVariant=InternalParameters  DVariant=InternalParameters  IntegratorVariant=Discrete  SatVariant=Enabled  AWVariant=Passthrough  PCopyVariant=Disabled  TRVariant=Disabled  FdbkBlocksVariant=Forward  IdealPFdbkVariant=Disabled  SatFdbkVariant=Disabled  DerivativeFilterVariant=ForwardEulerFilter  NVariant=InternalParameters  NCopyVariant=Disabled  FilterICVariant=InternalICsFilter  IntegratorICVariant=InternalICs  ExternalResetVariant=Disabled  TRSumVariant=Passthrough  SumFdbkVariant=Disabled  SumVariant=Sum_PID  TsampFilterVariant=InternalTs  TsampNgainVariant=Passthrough  TsampIntegralVariant=Disabled_SignalSpec  ExternalSaturationOutDataTypeStr=Inherit: Same as second input  DerivativeSourceVariant=ErrorSignal  PreIntVariant=InternalPreInt
  PMSM : Subsystem
  Product : Product
  Step : Step  Time=0.1  After=1000  SampleTime=0
  Sum : Sum  Inputs=++|
  Sum1 : Sum  Inputs=|+-
  Sum2 : Sum  Inputs=|++
  Sum3 : Sum  Inputs=|-+
  Sum4 : Sum  Inputs=++|
  Switch : Switch  Criteria=u2 > Threshold  SaturateOnIntegerOverflow=off  InputSameDT=off
  Switch1 : Switch  Criteria=u2 > Threshold  SaturateOnIntegerOverflow=off  InputSameDT=off
  Switch3 : Switch  Criteria=u2 > Threshold  SaturateOnIntegerOverflow=off  InputSameDT=off
  advanced firing angle : Constant  Value=theta_v
  control delay : Step  Time=2  SampleTime=0
  controller_1 : MATLAB Function  TreatAsAtomicUnit=on
  convert to mech speed : Gain  Gain=(2/P)*60/(2*pi)
  filter_enable : Step  Time=0.5  SampleTime=0
  hall sensors : MATLAB Function  TreatAsAtomicUnit=on
  hall_filter : Subsystem
  low_pass filter : TransferFcn  Denominator=[0.02 1]
  power_stage : Subsystem
  powergui1 : sps_lib/powergui  Priority=1  SimulationMode=Discrete  SampleTime=1e-6  frequency=60  Iterations=50  frequencyindice=0  Pbase=100e6  ErrMax=1e-4  UnitsV=kV  UnitsW=MW  buscounter=0  FunctionMessages=off  echomessages=off  EnableUseOfTLC=off  CurrentSourceSwitches=off  DisableSnubberDevices=off  DisableRonSwitches=off  DisableVfSwitches=off  DisplayEquations=off  AutomaticDiscreteSolvers=off  SolverType=Tustin/Backward Euler (TBE)  Interpol=off  ExternalGateDelay=off  methode=off  Ts=100  x0status=blocks  SPID=on  SwTol=0  HookPort=off  NonlinearTolerance=1e-4  nMaxIteration=100  ContinueOnMaxIteration=off  RestoreLinks=warning  ResistiveCurrentMeasurement=off  Frange=[0:2:500]  Ylog=off  Xlog=on  ShowGrid=off  save=off  variable=ZData  structure=0  ZoomFFT=off  StartTime=0.0  cycles=1  DisplayStyle=1  fundamental=60  FreqAxis=off  MaxFrequency=1000  frequencyindicesteady=1  RmsSteady=1  display=off
  qd-frame to stator : MATLAB Function  TreatAsAtomicUnit=on
  speed scope 120 : Scope  NumInputPorts=2
      settings: ActiveDisplayYMinimum=-1.1385486491945782E+15  ActiveDisplayYMaximum=1.0246937842751196E+16  DataLoggingVariableName=ScopeData5
  stator to qd-frame : MATLAB Function  TreatAsAtomicUnit=on
  torque ref [Nm] : Step  Time=0.1  After=1e-1  SampleTime=0  ZeroCross=off
  torque ref [Nm]1 : Step  After=-0.5e-1  SampleTime=0
  torque scope 120 : Scope  NumInputPorts=2
      settings: ActiveDisplayYMinimum=-0.89883  ActiveDisplayYMaximum=8.08945  DataLoggingVariableName=ScopeData6
  f_Hz : Outport
  i_ds_avs [A] : Outport  Port=2
  i_ds [A] : Outport  Port=3
  i_a [A] : Outport  Port=4
  i_b [A] : Outport  Port=5
  i_c [A] : Outport  Port=6
  electrical torque (T_e) [Nm] : Outport  Port=7
  e_q : Outport  Port=8
  hall_errors : Outport  Port=9
  rotor speed [rpm] : Outport  Port=10
  duty cycle : Outport  Port=11
  wires:
  Sum1/1 -> PID Controller/1
  Sum3/1 -> Gain/1
  power_stage/1(v_a) -> stator to qd-frame/1(fa)  "v_as"
  hall sensors/3(H3) -> [H3]
  qd-frame to stator/1(fa) -> i_a [A]/1, power_stage/1(i_a)  "i_a"
  convert to mech speed/1 -> rotor speed [rpm]/1, Switch1/1, speed scope 120/2  "rotor speed"
  qd-frame to stator/2(fb) -> i_b [A]/1, power_stage/2(i_b)  "i_b"
  hall_filter/1(result_state) -> Switch3/1
  PMSM/3(omega_r) -> MATLAB Function1/1(omega_r), convert to mech speed/1, [omega_r], Integrator/1  "electrical speed (omega_r)"
  MATLAB Function/1(HALL_STATE) -> [hall_state], Switch3/3  "unfiltered_state"
  Constant6/1 -> Manual Switch1/2
  Sum2/1 -> torque scope 120/1, Switch/3  "torque ref"
  control delay/1 -> Product/2
  [H1] -> hall_filter/1(H1), MATLAB Function/1(H1)  "H1"
  Mech torque [Nm]/1 -> PMSM/3(T_m)
  Step/1 -> speed scope 120/1, Switch/1  "speed ref"
  Switch3/1 -> controller_1/1(HALL_STATE)  "result_state"
  PMSM/2(i_ds) -> i_ds [A]/1, qd-frame to stator/2(fd), Moving Average (Variable Frequency)/2  "i_ds"
  Constant/1 -> hall sensors/1(hall_errors)
  PMSM/1(i_qs) -> qd-frame to stator/1(fq)  "i_qs"
  [omega_r] -> low_pass filter/1  "omega_r"
  power_stage/2(v_b) -> stator to qd-frame/2(fb)  "v_bs"
  Constant1/1 -> power_stage/5(duty_cycle)
  Manual Switch1/1 -> Switch3/2, hall_filter/4(filter_enable)
  PID Controller1/1 -> [del_phi]  "del_phi"
  hall sensors/1(H1) -> [H1]
  1 = speed ctrl 0 = torque ctrl/1 -> Switch/2, Switch1/2
  PMSM/4(T_e) -> electrical torque (T_e) [Nm]/1, torque scope 120/2, Switch1/3  "T_e"
  Moving Average (Variable Frequency)/1 -> i_ds_avs [A]/1, Product/1
  [H2] -> hall_filter/2(H2), MATLAB Function/2(H2)
  PMSM/5(e_q) -> e_q/1
  MATLAB Function1/1(f_Hz) -> Gain1/1
  torque ref [Nm]/1 -> Sum2/1  "torque ref"
  hall sensors/2(H2) -> [H2]
  Sum4/1 -> hall sensors/2(theta_r)
  Gain/1 -> PID Controller1/1
  filter_enable/1 -> Manual Switch1/1
  low_pass filter/1 -> hall_filter/5(omega_e)
  Constant3/1 -> hall_errors/1  "hall_errors"
  power_stage/3(v_c) -> stator to qd-frame/3(fc)  "v_cs"
  [del_phi] -> Sum4/1
  qd-frame to stator/3(fc) -> i_c [A]/1, power_stage/3(i_c)  "i_c"
  torque ref [Nm]1/1 -> Sum2/2  "torque ref"
  Switch1/1 -> Sum1/2
  Product/1 -> Sum3/1
  Integrator/1 -> stator to qd-frame/4(theta), Sum/2, qd-frame to stator/3(theta)  "theta_r"
  PID Controller/1 -> duty cycle/1  "duty cycle"
  Constant4/1 -> Sum3/2
  Gain1/1 -> f_Hz/1, Moving Average (Variable Frequency)/1
  stator to qd-frame/1(fq) -> PMSM/1(vq)  "v_qs"
  Sum/1 -> Sum4/2
  Switch/1 -> Sum1/1
  [H3] -> hall_filter/3(H3), MATLAB Function/3(H3)
  advanced firing angle/1 -> Sum/1
  stator to qd-frame/2(fd) -> PMSM/2(vd)  "v_ds"
  controller_1/1(T_vec) -> power_stage/4(T_vec)

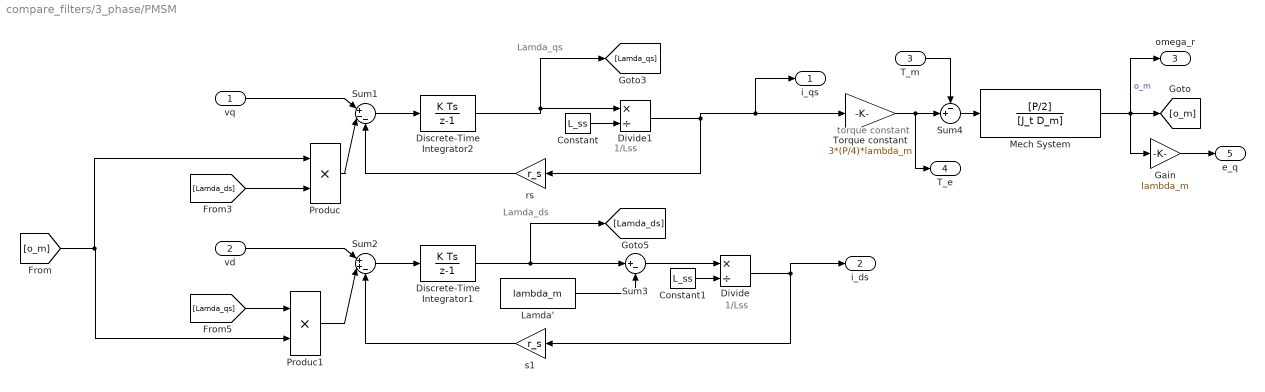
== system compare_filters/3_phase/PMSM ==
  note: torque constant
  note: Lamda_ds
  note: Lamda_qs
  note: 1/Lss
  note: 1/Lss
  vq : Inport
  vd : Inport  Port=2
  T_m : Inport  Port=3
  Constant : Constant  Value=L_ss
  Constant1 : Constant  Value=L_ss
  Discrete-Time Integrator1 : DiscreteIntegrator  SampleTime=-1  ICPrevOutput=DiscIntNeverNeededParam  ICPrevScaledInput=DiscIntNeverNeededParam
  Discrete-Time Integrator2 : DiscreteIntegrator  SampleTime=-1  ICPrevOutput=DiscIntNeverNeededParam  ICPrevScaledInput=DiscIntNeverNeededParam
  Divide : Product  Inputs=*/
  Divide1 : Product  Inputs=*/
  Gain : Gain  Gain=lambda_m
  Lamda' : Constant  Value=lambda_m
  Mech System : TransferFcn  Numerator=[P/2]  Denominator=[J_t D_m]
  Produc : Product  RndMeth=Zero
  Produc1 : Product  RndMeth=Zero
  Sum1 : Sum  Inputs=|+--
  Sum2 : Sum  Inputs=|++-
  Sum3 : Sum  Inputs=|+-
  Sum4 : Sum  Inputs=-+|
  Torque constant : Gain  Gain=3*(P/4)*lambda_m
  rs : Gain  Gain=r_s
  s1 : Gain  Gain=r_s
  i_qs : Outport
  i_ds : Outport  Port=2
  omega_r : Outport  Port=3
  T_e : Outport  Port=4
  e_q : Outport  Port=5
  wires:
  vd/1 -> Sum2/1
  vq/1 -> Sum1/1
  [Lamda_qs] -> Produc1/1
  [Lamda_ds] -> Produc/2
  [o_m] -> Produc1/2, Produc/1
  Lamda'/1 -> Sum3/2
  Sum3/1 -> Divide/1
  s1/1 -> Sum2/3
  Discrete-Time Integrator1/1 -> [Lamda_ds], Sum3/1
  Sum2/1 -> Discrete-Time Integrator1/1
  Produc1/1 -> Sum2/2
  Divide1/1 -> i_qs/1, Torque constant/1, rs/1
  rs/1 -> Sum1/3
  Discrete-Time Integrator2/1 -> [Lamda_qs], Divide1/1
  Sum1/1 -> Discrete-Time Integrator2/1
  Produc/1 -> Sum1/2
  Torque constant/1 -> Sum4/2, T_e/1
  Divide/1 -> i_ds/1, s1/1
  T_m/1 -> Sum4/1
  Sum4/1 -> Mech System/1
  Constant/1 -> Divide1/2
  Constant1/1 -> Divide/2
  Mech System/1 -> Gain/1, omega_r/1, [o_m]  "o_m"
  Gain/1 -> e_q/1

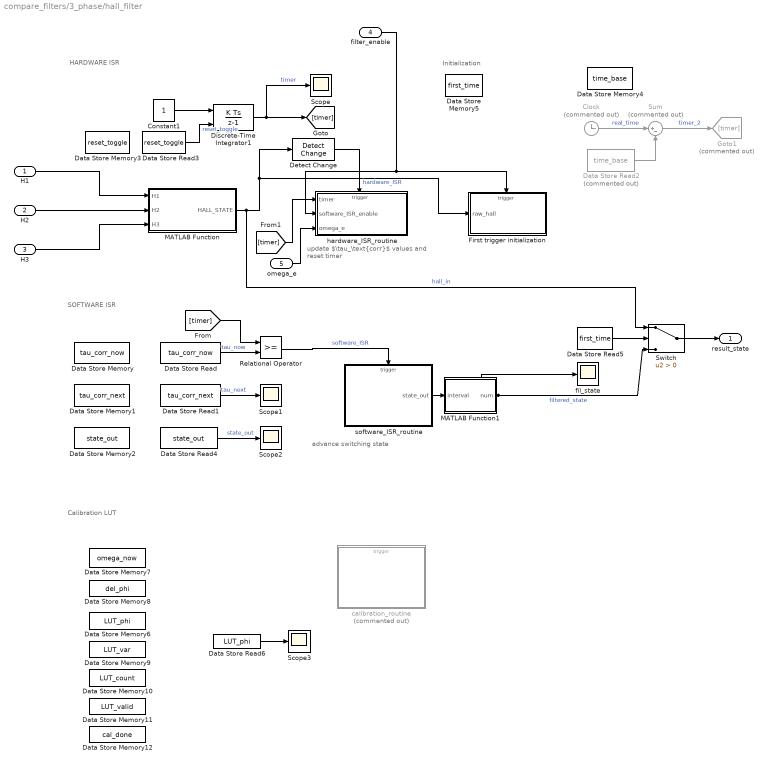
== system compare_filters/3_phase/hall_filter ==
  note: Calibration LUT
  note: Initialization
  note: SOFTWARE ISR
  note: HARDWARE ISR
  note: update $\tau_\text{corr}$ values and reset timer
  note: advance switching state
  H1 : Inport
  H2 : Inport  Port=2
  H3 : Inport  Port=3
  filter_enable : Inport  Port=4
  omega_e : Inport  Port=5
  Clock : Clock  Commented=on
  Constant1 : Constant
  Data Store Memory : DataStoreMemory  DataStoreName=tau_corr_now  WriteAfterWriteMsg=warning  InitialValue=-1  ShowAdditionalParam=off
  Data Store Memory1 : DataStoreMemory  DataStoreName=tau_corr_next  WriteAfterWriteMsg=warning  InitialValue=-1  ShowAdditionalParam=off
  Data Store Memory10 : DataStoreMemory  DataStoreName=LUT_count  WriteAfterWriteMsg=warning  InitialValue=[0 0 0 0 0 0]  ShowAdditionalParam=off
  Data Store Memory11 : DataStoreMemory  DataStoreName=LUT_valid  WriteAfterWriteMsg=warning  InitialValue=[0 0 0 0 0 0]  ShowAdditionalParam=off
  Data Store Memory12 : DataStoreMemory  DataStoreName=cal_done  WriteAfterWriteMsg=warning  ShowAdditionalParam=off  OutDataTypeStr=boolean
  Data Store Memory2 : DataStoreMemory  DataStoreName=state_out  WriteAfterWriteMsg=warning  InitialValue=2  ShowAdditionalParam=off
  Data Store Memory3 : DataStoreMemory  DataStoreName=reset_toggle  WriteAfterWriteMsg=warning  ShowAdditionalParam=off
  Data Store Memory4 : DataStoreMemory  DataStoreName=time_base  WriteAfterWriteMsg=warning  ShowAdditionalParam=off
  Data Store Memory5 : DataStoreMemory  DataStoreName=first_time  WriteAfterWriteMsg=warning  InitialValue=1  ShowAdditionalParam=off
  Data Store Memory6 : DataStoreMemory  DataStoreName=LUT_phi  WriteAfterWriteMsg=warning  InitialValue=[0 0 0 0 0 0]  ShowAdditionalParam=off
  Data Store Memory7 : DataStoreMemory  DataStoreName=omega_now  WriteAfterWriteMsg=warning  ShowAdditionalParam=off
  Data Store Memory8 : DataStoreMemory  DataStoreName=del_phi  WriteAfterWriteMsg=warning  ShowAdditionalParam=off
  Data Store Memory9 : DataStoreMemory  DataStoreName=LUT_var  WriteAfterWriteMsg=warning  InitialValue=[0 0 0 0 0 0]  ShowAdditionalParam=off
  Data Store Read : DataStoreRead  DataStoreName=tau_corr_now  IndexOptions=Index vector (dialog)  Indices=1  OutputSizes=1
  Data Store Read1 : DataStoreRead  DataStoreName=tau_corr_next  IndexOptions=Index vector (dialog)  Indices=1  OutputSizes=1
  Data Store Read2 : DataStoreRead  Commented=on  DataStoreName=time_base  IndexOptions=Index vector (dialog)  Indices=1  OutputSizes=1
  Data Store Read3 : DataStoreRead  DataStoreName=reset_toggle  IndexOptions=Index vector (dialog)  Indices=1  OutputSizes=1
  Data Store Read4 : DataStoreRead  DataStoreName=state_out  IndexOptions=Index vector (dialog)  Indices=1  OutputSizes=1
  Data Store Read5 : DataStoreRead  DataStoreName=first_time  IndexOptions=Index vector (dialog)  Indices=1  OutputSizes=1
  Data Store Read6 : DataStoreRead  DataStoreName=LUT_phi  IndexOptions=Index vector (dialog)  Indices=1  OutputSizes=1
  Detect Change : simulink/Logic and Bit Operations/Detect Change  vinit=0  OutDataTypeStr=boolean
  Discrete-Time Integrator1 : DiscreteIntegrator  ExternalReset=either  SampleTime=1/(1e6)  ICPrevOutput=DiscIntNeverNeededParam  ICPrevScaledInput=DiscIntNeverNeededParam
  First trigger initialization : Subsystem  TreatAsAtomicUnit=on
  Goto1 : Goto  Commented=on  GotoTag=timer
  MATLAB Function : MATLAB Function  TreatAsAtomicUnit=on
  MATLAB Function1 : MATLAB Function  TreatAsAtomicUnit=on
  Relational Operator : RelationalOperator  OutDataTypeStr=boolean  RndMeth=Simplest  InputSameDT=off
  Scope{,1..3} (4 alike) : Scope
      Scope settings: ActiveDisplayYMinimum=-6.25  ActiveDisplayYMaximum=56.25
      Scope1 settings: ActiveDisplayYMinimum=7.96701  ActiveDisplayYMaximum=8.03137
      Scope2 settings: ActiveDisplayYMinimum=7.96701  ActiveDisplayYMaximum=8.03137
      Scope3 settings: ActiveDisplayYMinimum=0.99241576103971962  ActiveDisplayYMaximum=1.0799572702760518  DataLoggingVariableName=ScopeData2
  Sum : Sum  Commented=on  Inputs=|+-
  Switch : Switch  Criteria=u2 > Threshold  SaturateOnIntegerOverflow=off  InputSameDT=off
  calibration_routine : Subsystem  Priority=11  Commented=on  TreatAsAtomicUnit=on
  fil_state : Scope
      settings: ActiveDisplayYMinimum=-0.75  ActiveDisplayYMaximum=6.75  DataLoggingVariableName=ScopeData3
  hardware_ISR_routine : Subsystem  Priority=1
  software_ISR_routine : Subsystem  Priority=10  TreatAsAtomicUnit=on
  result_state : Outport
  wires:
  Discrete-Time Integrator1/1 -> [timer], Scope/1  "timer"
  Relational Operator/1 -> software_ISR_routine/Trigger  "software_ISR"
  Constant1/1 -> Discrete-Time Integrator1/1
  [timer] -> Relational Operator/1
  software_ISR_routine/1(state_out) -> MATLAB Function1/1(interval)
  MATLAB Function/1(HALL_STATE) -> Switch/1, Detect Change/1, First trigger initialization/1(raw_hall)  "hall_in"
  Data Store Read3/1 -> Discrete-Time Integrator1/2  "reset_toggle"
  Data Store Read1/1 -> Scope1/1  "tau_next"
  Data Store Read/1 -> Relational Operator/2  "tau_now"
  H3/1 -> MATLAB Function/3(H3)
  H2/1 -> MATLAB Function/2(H2)
  H1/1 -> MATLAB Function/1(H1)
  MATLAB Function1/1(num) -> fil_state/1, Switch/3  "filtered_state"
  Detect Change/1 -> hardware_ISR_routine/Trigger  "hardware_ISR"
  Data Store Read4/1 -> Scope2/1  "state_out"
  filter_enable/1 -> First trigger initialization/Trigger, hardware_ISR_routine/2(software_ISR_enable)
  Clock/1 -> Sum/1  "real_time"
  [timer] -> hardware_ISR_routine/1(timer)
  Data Store Read2/1 -> Sum/2
  Sum/1 -> Goto1/1  "timer_2"
  Data Store Read5/1 -> Switch/2
  Switch/1 -> result_state/1
  Data Store Read6/1 -> Scope3/1
  omega_e/1 -> hardware_ISR_routine/3(omega_e)
